simulink library "autolibbatterycommon"  (R2019b)
settings: Solver=ode45  StartTime=0.0  StopTime=10.0  RelTol=1e-3  EnableMultiTasking=on
undefined symbols (not defined in the file or in its folder): BattCap, BattCapInit, BattChargeMax, BattTempBp, C, C1, C2, C3, C4, C5, Cap_LUT, CapacityAh, CapLUTBp, CapSOCBp, CapVolt, Current_BP, DiscIntNeverNeededParam, Em, InitialCapVoltage, InitialChargeRemAh, Np, Ns, R, R0, R1, R2, R3, R4, R5, RefBlkName, RInt, SOC_BP, T1, Tc, Temp_BP, Temperature_BP, Ts, Vinit, Vu
libraries: $bdroot x72, autolibpowerinfoutils x1
(part 2 of 2)

== system autolibbatterycommon/5RC/Voltage ==
  Em : Inport
  R0 : Inport  Port=2
  BattAmp : Inport  Port=3
  RC1 : Inport  Port=4
  RC2 : Inport  Port=5
  RC3 : Inport  Port=6
  RC4 : Inport  Port=7
  RC5 : Inport  Port=8
  Add : Sum  Inputs=+------
  Product : Product
  BattVolt : Outport  VectorParamsAs1DForOutWhenUnconnected=off
  wires:
  RC4/1 -> Add/6
  RC2/1 -> Add/4
  RC1/1 -> Add/3
  Add/1 -> BattVolt/1
  RC3/1 -> Add/5
  Em/1 -> Add/1
  Product/1 -> Add/2
  R0/1 -> Product/1
  RC5/1 -> Add/7
  BattAmp/1 -> Product/2

== system autolibbatterycommon/CoreBattery/Charge Model ==
  LdAmp : Inport
  Gain1 : Gain  Gain=-1/(Np*3600)
  Integrator Limited : Integrator  InitialCondition=BattCapInit  LimitOutput=on  UpperSaturationLimit=BattChargeMax  LowerSaturationLimit=0
  LdAmpHr : Outport  VectorParamsAs1DForOutWhenUnconnected=off
  wires:
  Gain1/1 -> Integrator Limited/1
  Integrator Limited/1 -> LdAmpHr/1
  LdAmp/1 -> Gain1/1

== system autolibbatterycommon/CoreBattery/State of Charge Capacity ==
  LdAmpHr : Inport
  Constant1 : Constant  Value=BattChargeMax
  Divide : Product  Inputs=*/
  CapSOC : Outport  VectorParamsAs1DForOutWhenUnconnected=off
  wires:
  Constant1/1 -> Divide/2
  LdAmpHr/1 -> Divide/1
  Divide/1 -> CapSOC/1

== system autolibbatterycommon/CoreBattery/Subsystem ==
  CapSOC : Inport
  LdAmp : Inport  Port=2
  BattTemp : Inport  Port=3
  Em : Lookup_n-D  NumberOfTableDimensions=1  LookupTableObject=''  BreakpointsForDimension1=CapLUTBp  BreakpointsForDimension2=CapSOCBp  Table=Em  ExtrapMethod=Clip  UseLastTableValue=on  InternalRulePriority=Speed  RndMeth=Simplest  InputSameDT=on
  Gain1 : Gain  Gain=Ns
  Product : Product
  R : Lookup_n-D  LookupTableObject=''  BreakpointsForDimension1=BattTempBp  BreakpointsForDimension2=CapSOCBp  Table=RInt  ExtrapMethod=Clip  UseLastTableValue=on  InternalRulePriority=Speed  RndMeth=Simplest  InputSameDT=on
  Subtract : Sum  Inputs=+-
  OutVolt : Outport  VectorParamsAs1DForOutWhenUnconnected=off
  wires:
  Gain1/1 -> OutVolt/1
  Em/1 -> Subtract/1
  R/1 -> Product/1
  Product/1 -> Subtract/2
  BattTemp/1 -> R/1
  Subtract/1 -> Gain1/1
  LdAmp/1 -> Product/2
  CapSOC/1 -> Em/1, R/2

== system autolibbatterycommon/Datasheet Battery/Charge Model ==
  LdAmp : Inport
  CapInit : Inport  Port=2
  Constant1 : Constant  Value=BattChargeMax
  Gain1 : Gain  Gain=-1/(Np*3600)
  Integrator Limited : Integrator  InitialConditionSource=external  InitialCondition=BattCapInit  LimitOutput=on  UpperSaturationLimit=BattChargeMax  LowerSaturationLimit=0
  Switch : Switch  Criteria=u2 > Threshold  Threshold=BattChargeMax
  LdAmpHr : Outport  VectorParamsAs1DForOutWhenUnconnected=off
  wires:
  Gain1/1 -> Integrator Limited/1
  Integrator Limited/1 -> LdAmpHr/1
  LdAmp/1 -> Gain1/1
  CapInit/1 -> Switch/3, Switch/2
  Constant1/1 -> Switch/1
  Switch/1 -> Integrator Limited/2

== system autolibbatterycommon/Datasheet Battery/State of Charge Capacity ==
  LdAmpHr : Inport
  Constant1 : Constant  Value=BattChargeMax
  Divide : Product  Inputs=*/
  CapSOC : Outport  VectorParamsAs1DForOutWhenUnconnected=off
  wires:
  Constant1/1 -> Divide/2
  LdAmpHr/1 -> Divide/1
  Divide/1 -> CapSOC/1

== system autolibbatterycommon/Datasheet Battery/Voltage and Power Calculation ==
  CapSOC : Inport
  LdAmp : Inport  Port=2
  BattTemp : Inport  Port=3
  Em : Lookup_n-D  NumberOfTableDimensions=1  LookupTableObject=''  BreakpointsForDimension1=CapLUTBp  BreakpointsForDimension2=CapSOCBp  Table=Em  ExtrapMethod=Clip  UseLastTableValue=on  InternalRulePriority=Speed  RndMeth=Simplest  InputSameDT=on
  Gain1 : Gain  Gain=Ns
  Gain2 : Gain  Gain=1/Np
  Gain3 : Gain  Gain=Ns
  Gain4 : Gain  Gain=Np
  Product : Product
  Product1 : Product
  R : Lookup_n-D  LookupTableObject=''  BreakpointsForDimension1=BattTempBp  BreakpointsForDimension2=CapSOCBp  Table=RInt  ExtrapMethod=Clip  UseLastTableValue=on  InternalRulePriority=Speed  RndMeth=Simplest  InputSameDT=on
  Subtract : Sum  Inputs=+-
  OutVolt : Outport  VectorParamsAs1DForOutWhenUnconnected=off
  BattPwrLoss : Outport  Port=2  VectorParamsAs1DForOutWhenUnconnected=off
  wires:
  Gain1/1 -> OutVolt/1
  Em/1 -> Subtract/1
  R/1 -> Product/1
  Product/1 -> Product1/1, Subtract/2
  BattTemp/1 -> R/1
  Subtract/1 -> Gain1/1
  LdAmp/1 -> Gain2/1
  CapSOC/1 -> Em/1, R/2
  Gain2/1 -> Product1/2, Product/2
  Product1/1 -> Gain3/1
  Gain3/1 -> Gain4/1
  Gain4/1 -> BattPwrLoss/1

== system autolibbatterycommon/nRC_Battery_Core/1RC ==
  Current : Inport
  1-D Lookup Table : Lookup_n-D  NumberOfTableDimensions=4  LookupTableObject=''  BreakpointsForDimension1=SOC_BP  BreakpointsForDimension2=Current_BP  UseOneInputPortForAllInputData=on  Table=Em'  ExtrapMethod=Clip  UseLastTableValue=on  InternalRulePriority=Speed  RndMeth=Simplest  InputSameDT=on
  1-D Lookup Table1 : Lookup_n-D  LookupTableObject=''  BreakpointsForDimension1=SOC_BP  BreakpointsForDimension2=Current_BP  UseOneInputPortForAllInputData=on  Table=R0'  ExtrapMethod=Clip  UseLastTableValue=on  InternalRulePriority=Speed  RndMeth=Simplest  InputSameDT=on
  Add : Sum  Inputs=+++
  Product : Product
  RC1 : $bdroot/RC1  R=R1  C=C  SOC_BP=SOC_BP  Temperature_BP=Temp_BP  V_init=InitialCapVoltage(1)  V_upper=Vu  V_lower=Vl
  SOC Counter : $bdroot/SOC Counter  Q_init=InitialChargeRemAh  Cap=CapacityAh  Cap_LUT=Cap_LUT  Temp_BP=Temperature_BP
  Vector Concatenate : Concatenate
  SOC : Outport  VectorParamsAs1DForOutWhenUnconnected=off
  Voltage : Outport  Port=2  VectorParamsAs1DForOutWhenUnconnected=off
  wires:
  SOC Counter/1 -> SOC/1, Vector Concatenate/1
  RC1/1 -> Add/3
  Product/1 -> Add/2
  1-D Lookup Table1/1 -> Product/1
  Current/1 -> SOC Counter/1, Vector Concatenate/2, Product/2, RC1/2
  1-D Lookup Table/1 -> Add/1
  Vector Concatenate/1 -> RC1/1, 1-D Lookup Table1/1, 1-D Lookup Table/1
  Add/1 -> Voltage/1

== system autolibbatterycommon/nRC_Battery_Core/2RC ==
  Current : Inport
  1-D Lookup Table : Lookup_n-D  NumberOfTableDimensions=4  LookupTableObject=''  BreakpointsForDimension1=SOC_BP  BreakpointsForDimension2=Current_BP  UseOneInputPortForAllInputData=on  Table=Em'  ExtrapMethod=Clip  UseLastTableValue=on  InternalRulePriority=Speed  RndMeth=Simplest  InputSameDT=on
  1-D Lookup Table1 : Lookup_n-D  LookupTableObject=''  BreakpointsForDimension1=SOC_BP  BreakpointsForDimension2=Current_BP  UseOneInputPortForAllInputData=on  Table=R0'  ExtrapMethod=Clip  UseLastTableValue=on  InternalRulePriority=Speed  RndMeth=Simplest  InputSameDT=on
  Add : Sum  Inputs=++++
  Product : Product
  RC1 : $bdroot/RC1  R=R1  C=C  SOC_BP=SOC_BP  Temperature_BP=Temp_BP  V_init=InitialCapVoltage(1)  V_upper=Vu  V_lower=Vl
  RC2 : $bdroot/RC1  R=R2  C=C  SOC_BP=SOC_BP  Temperature_BP=Temp_BP  V_init=InitialCapVoltage(2)  V_upper=Vu  V_lower=Vl
  SOC Counter : $bdroot/SOC Counter  Q_init=InitialChargeRemAh  Cap=CapacityAh  Cap_LUT=Cap_LUT  Temp_BP=Temperature_BP
  Vector Concatenate : Concatenate
  SOC : Outport  VectorParamsAs1DForOutWhenUnconnected=off
  Voltage : Outport  Port=2  VectorParamsAs1DForOutWhenUnconnected=off
  wires:
  Vector Concatenate/1 -> 1-D Lookup Table/1, 1-D Lookup Table1/1, RC2/1, RC1/1
  1-D Lookup Table/1 -> Add/1
  Add/1 -> Voltage/1
  Current/1 -> SOC Counter/1, RC2/2, RC1/2, Product/2, Vector Concatenate/2
  1-D Lookup Table1/1 -> Product/1
  Product/1 -> Add/2
  RC1/1 -> Add/3
  RC2/1 -> Add/4
  SOC Counter/1 -> Vector Concatenate/1, SOC/1

== system autolibbatterycommon/nRC_Battery_Core/3RC ==
  Current : Inport
  1-D Lookup Table : Lookup_n-D  LookupTableObject=''  BreakpointsForDimension1=SOC_BP  BreakpointsForDimension2=Current_BP  UseOneInputPortForAllInputData=on  Table=Em  ExtrapMethod=Clip  UseLastTableValue=on  InternalRulePriority=Speed  RndMeth=Simplest  InputSameDT=on
  1-D Lookup Table1 : Lookup_n-D  LookupTableObject=''  BreakpointsForDimension1=SOC_BP  BreakpointsForDimension2=Current_BP  UseOneInputPortForAllInputData=on  Table=R0  ExtrapMethod=Clip  UseLastTableValue=on  InternalRulePriority=Speed  RndMeth=Simplest  InputSameDT=on
  Add : Sum  Inputs=+++++
  Product : Product
  RC1 : $bdroot/RC1  R=R1  C=C  SOC_BP=SOC_BP  Temperature_BP=Temp_BP  V_init=InitialCapVoltage(1)  V_upper=Vu  V_lower=Vl
  RC2 : $bdroot/RC1  R=R2  C=C  SOC_BP=SOC_BP  Temperature_BP=Temp_BP  V_init=InitialCapVoltage(2)  V_upper=Vu  V_lower=Vl
  RC3 : $bdroot/RC1  R=R3  C=C  SOC_BP=SOC_BP  Temperature_BP=Temp_BP  V_init=InitialCapVoltage(3)  V_upper=Vu  V_lower=Vl
  SOC Counter : $bdroot/SOC Counter  Q_init=InitialChargeRemAh  Cap=CapacityAh  Cap_LUT=Cap_LUT  Temp_BP=Temp_BP
  Vector Concatenate : Concatenate
  SOC : Outport  VectorParamsAs1DForOutWhenUnconnected=off
  Voltage : Outport  Port=2  VectorParamsAs1DForOutWhenUnconnected=off
  wires:
  SOC Counter/1 -> SOC/1, Vector Concatenate/1
  RC3/1 -> Add/5
  RC2/1 -> Add/4
  RC1/1 -> Add/3
  Product/1 -> Add/2
  1-D Lookup Table1/1 -> Product/1
  Current/1 -> SOC Counter/1, Vector Concatenate/2, Product/2, RC1/2, RC3/2, RC2/2
  Add/1 -> Voltage/1
  1-D Lookup Table/1 -> Add/1
  Vector Concatenate/1 -> RC1/1, RC3/1, RC2/1, 1-D Lookup Table1/1, 1-D Lookup Table/1

== system autolibbatterycommon/nRC_Battery_Core/4RC ==
  Current : Inport
  1-D Lookup Table : Lookup_n-D  NumberOfTableDimensions=4  LookupTableObject=''  BreakpointsForDimension1=SOC_BP  BreakpointsForDimension2=Current_BP  UseOneInputPortForAllInputData=on  Table=Em'  ExtrapMethod=Clip  UseLastTableValue=on  InternalRulePriority=Speed  RndMeth=Simplest  InputSameDT=on
  1-D Lookup Table1 : Lookup_n-D  LookupTableObject=''  BreakpointsForDimension1=SOC_BP  BreakpointsForDimension2=Current_BP  UseOneInputPortForAllInputData=on  Table=R0'  ExtrapMethod=Clip  UseLastTableValue=on  InternalRulePriority=Speed  RndMeth=Simplest  InputSameDT=on
  Add : Sum  Inputs=++++++
  Product : Product
  RC1 : $bdroot/RC1  R=R1  C=C  SOC_BP=SOC_BP  Temperature_BP=Temp_BP  V_init=InitialCapVoltage(1)  V_upper=Vu  V_lower=Vl
  RC2 : $bdroot/RC1  R=R2  C=C  SOC_BP=SOC_BP  Temperature_BP=Temp_BP  V_init=InitialCapVoltage(2)  V_upper=Vu  V_lower=Vl
  RC3 : $bdroot/RC1  R=R3  C=C  SOC_BP=SOC_BP  Temperature_BP=Temp_BP  V_init=InitialCapVoltage(3)  V_upper=Vu  V_lower=Vl
  RC4 : $bdroot/RC1  R=R4  C=C  SOC_BP=SOC_BP  Temperature_BP=Temp_BP  V_init=InitialCapVoltage(4)  V_upper=Vu  V_lower=Vl
  SOC Counter : $bdroot/SOC Counter  Q_init=InitialChargeRemAh  Cap=CapacityAh  Cap_LUT=Cap_LUT  Temp_BP=Temperature_BP
  Vector Concatenate : Concatenate
  SOC : Outport  VectorParamsAs1DForOutWhenUnconnected=off
  Voltage : Outport  Port=2  VectorParamsAs1DForOutWhenUnconnected=off
  wires:
  Vector Concatenate/1 -> 1-D Lookup Table/1, 1-D Lookup Table1/1, RC4/1, RC3/1, RC2/1, RC1/1
  1-D Lookup Table/1 -> Add/1
  Add/1 -> Voltage/1
  Current/1 -> SOC Counter/1, RC4/2, RC3/2, RC2/2, RC1/2, Product/2, Vector Concatenate/2
  1-D Lookup Table1/1 -> Product/1
  Product/1 -> Add/2
  RC1/1 -> Add/3
  RC2/1 -> Add/4
  RC3/1 -> Add/5
  SOC Counter/1 -> Vector Concatenate/1, SOC/1
  RC4/1 -> Add/6

== system autolibbatterycommon/nRC_Battery_Core/5RC ==
  Current : Inport
  1-D Lookup Table : Lookup_n-D  NumberOfTableDimensions=4  LookupTableObject=''  BreakpointsForDimension1=SOC_BP  BreakpointsForDimension2=Current_BP  UseOneInputPortForAllInputData=on  Table=Em'  ExtrapMethod=Clip  UseLastTableValue=on  InternalRulePriority=Speed  RndMeth=Simplest  InputSameDT=on
  1-D Lookup Table1 : Lookup_n-D  LookupTableObject=''  BreakpointsForDimension1=SOC_BP  BreakpointsForDimension2=Current_BP  UseOneInputPortForAllInputData=on  Table=R0'  ExtrapMethod=Clip  UseLastTableValue=on  InternalRulePriority=Speed  RndMeth=Simplest  InputSameDT=on
  Add : Sum  Inputs=+++++++
  Product : Product
  RC1 : $bdroot/RC1  R=R1  C=C  SOC_BP=SOC_BP  Temperature_BP=Temp_BP  V_init=InitialCapVoltage(1)  V_upper=Vu  V_lower=Vl
  RC2 : $bdroot/RC1  R=R2  C=C  SOC_BP=SOC_BP  Temperature_BP=Temp_BP  V_init=InitialCapVoltage(2)  V_upper=Vu  V_lower=Vl
  RC3 : $bdroot/RC1  R=R3  C=C  SOC_BP=SOC_BP  Temperature_BP=Temp_BP  V_init=InitialCapVoltage(3)  V_upper=Vu  V_lower=Vl
  RC4 : $bdroot/RC1  R=R4  C=C  SOC_BP=SOC_BP  Temperature_BP=Temp_BP  V_init=InitialCapVoltage(4)  V_upper=Vu  V_lower=Vl
  RC5 : $bdroot/RC1  R=R5  C=C  SOC_BP=SOC_BP  Temperature_BP=Temp_BP  V_init=InitialCapVoltage(5)  V_upper=Vu  V_lower=Vl
  SOC Counter : $bdroot/SOC Counter  Q_init=InitialChargeRemAh  Cap=CapacityAh  Cap_LUT=Cap_LUT  Temp_BP=Temperature_BP
  Vector Concatenate : Concatenate
  SOC : Outport  VectorParamsAs1DForOutWhenUnconnected=off
  Voltage : Outport  Port=2  VectorParamsAs1DForOutWhenUnconnected=off
  wires:
  SOC Counter/1 -> SOC/1, Vector Concatenate/1
  RC3/1 -> Add/5
  RC2/1 -> Add/4
  RC1/1 -> Add/3
  Product/1 -> Add/2
  1-D Lookup Table1/1 -> Product/1
  Current/1 -> SOC Counter/1, Vector Concatenate/2, Product/2, RC1/2, RC5/2, RC4/2, RC3/2, RC2/2
  Add/1 -> Voltage/1
  1-D Lookup Table/1 -> Add/1
  Vector Concatenate/1 -> RC1/1, RC2/1, RC5/1, RC4/1, RC3/1, 1-D Lookup Table1/1, 1-D Lookup Table/1
  RC5/1 -> Add/7
  RC4/1 -> Add/6
